simulink subsystem "quarter_car_w_tire_subsystem"  (R2020b)
settings: Solver=VariableStepAuto  StartTime=0.0  StopTime=10.0  RelTol=1e-3
settings Model: Creator=Ricky  LastModifiedBy=Ricky

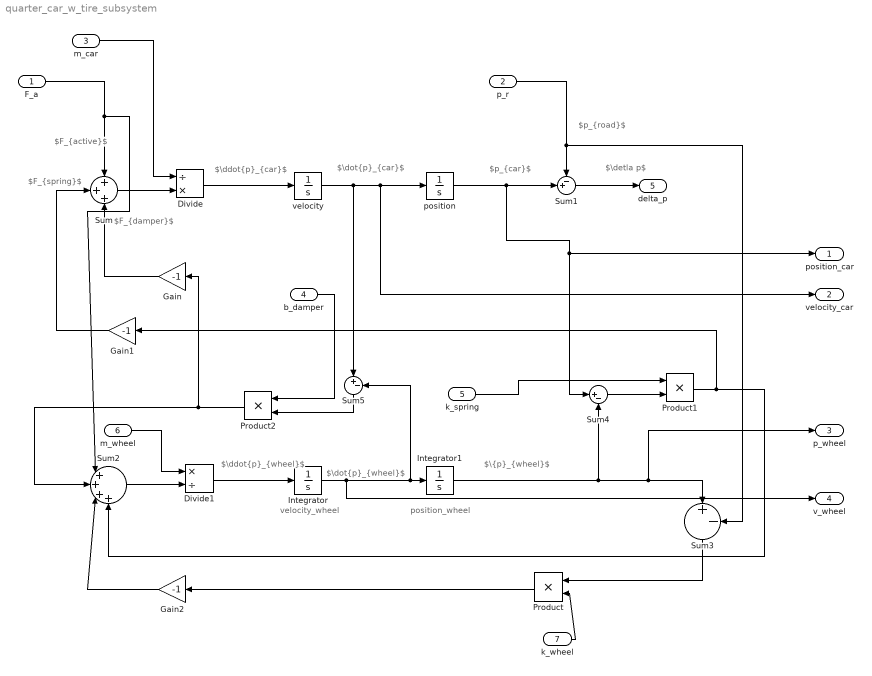
== system quarter_car_w_tire_subsystem ==
  note: $\dot{p}_{wheel}$
  note: position_wheel
  note: velocity_wheel
  note: $\ddot{p}_{wheel}$
  note: $\ddot{p}_{car}$
  note: $\detla p$
  note: $\dot{p}_{car}$
  note: $F_{active}$
  note: $p_{car}$
  note: $p_{road}$
  note: $F_{damper}$
  note: $F_{spring}$
  note: $\{p}_{wheel}$
  F_a : Inport
  p_r : Inport  Port=2
  m_car : Inport  Port=3
  b_damper : Inport  Port=4
  k_spring : Inport  Port=5
  m_wheel : Inport  Port=6
  k_wheel : Inport  Port=7
  Divide : Product  Inputs=/*
  Divide1 : Product  Inputs=*/
  Gain : Gain  Gain=-1
  Gain1 : Gain  Gain=-1
  Gain2 : Gain  Gain=-1
  Integrator : Integrator
  Integrator1 : Integrator
  Product : Product
  Product1 : Product
  Product2 : Product
  Sum : Sum  Inputs=+++
  Sum1 : Sum  Inputs=-+|
  Sum2 : Sum  Inputs=|++++
  Sum3 : Sum  Inputs=|+-
  Sum4 : Sum  Inputs=|+-
  Sum5 : Sum  Inputs=|+-
  position : Integrator
  velocity : Integrator
  position_car : Outport
  velocity_car : Outport  Port=2
  p_wheel : Outport  Port=3
  v_wheel : Outport  Port=4
  delta_p : Outport  Port=5
  wires:
  Gain1/1 -> Sum/2
  k_wheel/1 -> Product/2
  Gain/1 -> Sum/3
  Product/1 -> Gain2/1
  m_wheel/1 -> Divide1/1
  Divide1/1 -> Integrator/1
  Integrator1/1 -> Sum3/1, p_wheel/1, Sum4/2
  k_spring/1 -> Product1/1
  Divide/1 -> velocity/1
  Sum4/1 -> Product1/2
  Sum3/1 -> Product/1
  Gain2/1 -> Sum2/3
  Product1/1 -> Sum2/4, Gain1/1
  Sum2/1 -> Divide1/2
  Sum5/1 -> Product2/2
  position/1 -> Sum1/2, Sum4/1, position_car/1
  Sum/1 -> Divide/2
  b_damper/1 -> Product2/1
  Product2/1 -> Sum2/2, Gain/1
  m_car/1 -> Divide/1
  p_r/1 -> Sum1/1, Sum3/2
  F_a/1 -> Sum/1, Sum2/1
  velocity/1 -> position/1, velocity_car/1, Sum5/1
  Sum1/1 -> delta_p/1
  Integrator/1 -> Integrator1/1, Sum5/2, v_wheel/1
